simulink model "lab_1_position_sim"  (R2018b)
settings: Solver=ode3  StartTime=0.0  StopTime=10.0  FixedStep=0.01  RelTol=1e-3
values from neighbouring files (symbols this model uses):
  K = K_alpha / alpha    [lab (3).m]    (also in lab (4).m; lab1.m = (omega_natural ^ 2) / (6 * K1 * amp * alpha))
  tau = (1 - (tau2 * alpha)) / (1 - (2 * z * w * tau2)) / alpha    [lab (3).m]    (also in lab (4).m; lab1.m = ((tau1 * alpha) - 1) / (alpha * ((2 * zeta * omega_natural *)
  tau2 = 0.08    [lab (3).m]    (also in lab (4).m)
undefined symbols (not defined in the file or in its folder): DiscIntNeverNeededParam, k1, k2
libraries: simulink x2
settings Model: Creator=MSI  LastModifiedBy=Oguz
settings OptimizationCC: LifeSpan=inf
settings CodeAppCC: StateflowObjectComments=on

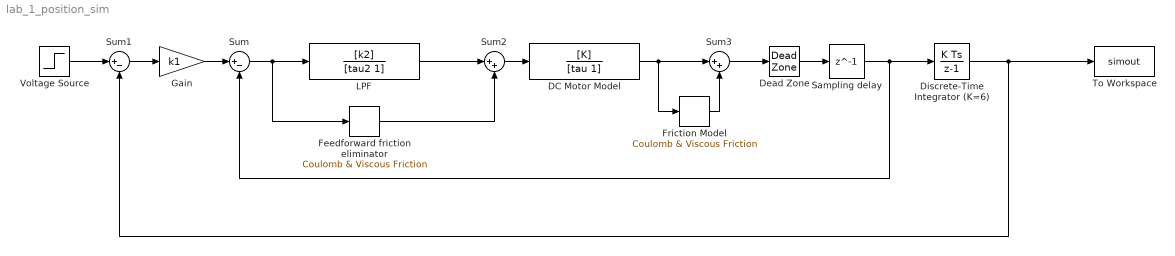
== system lab_1_position_sim ==
  DC Motor Model : TransferFcn  Numerator=[K]  Denominator=[tau 1]
  Dead Zone : DeadZone  LowerValue=-10  UpperValue=10  SaturateOnIntegerOverflow=on
  Discrete-Time Integrator (K=6) : DiscreteIntegrator  gainval=6  SampleTime=-1  ICPrevOutput=DiscIntNeverNeededParam  ICPrevScaledInput=DiscIntNeverNeededParam
  Feedforward friction eliminator : simulink/Discontinuities/Coulomb & Viscous Friction  offset=2  gain=0
      settings: SourceProductName=Simulink
  Friction Model : simulink/Discontinuities/Coulomb & Viscous Friction  offset=-15  gain=-0.1
      settings: SourceProductName=Simulink
  Gain : Gain  Gain=k1
  LPF : TransferFcn  Numerator=[k2]  Denominator=[tau2 1]
  Sampling delay : Delay  DelayLength=1
  Sum : Sum  Inputs=|+-
  Sum1 : Sum  Inputs=|+-
  Sum2 : Sum  Inputs=|++
  Sum3 : Sum  Inputs=|++
  To Workspace : ToWorkspace  VariableName=simout  SaveFormat=Timeseries  SampleTime=-1
  Voltage Source : Step  Time=0  After=90  SampleTime=0
  wires:
  Sum3/1 -> Dead Zone/1
  LPF/1 -> Sum2/1
  Sum1/1 -> Gain/1
  Sum2/1 -> DC Motor Model/1
  Discrete-Time Integrator (K=6)/1 -> To Workspace/1, Sum1/2
  Sum/1 -> Feedforward friction eliminator/1, LPF/1
  DC Motor Model/1 -> Friction Model/1, Sum3/1
  Friction Model/1 -> Sum3/2
  Feedforward friction eliminator/1 -> Sum2/2
  Gain/1 -> Sum/1
  Voltage Source/1 -> Sum1/1
  Dead Zone/1 -> Sampling delay/1
  Sampling delay/1 -> Discrete-Time Integrator (K=6)/1, Sum/2
